simulink model "Mackey-Glass"  (R2020b)
settings: Solver=FixedStepAuto  StartTime=0.0  StopTime=TFinal  FixedStep=0.001  RelTol=1e-3
undefined symbols (not defined in the file or in its folder): coupling, decay_rate, n, nodes
libraries: simulink x1
settings Model: Creator=tian  LastModifiedBy=tian

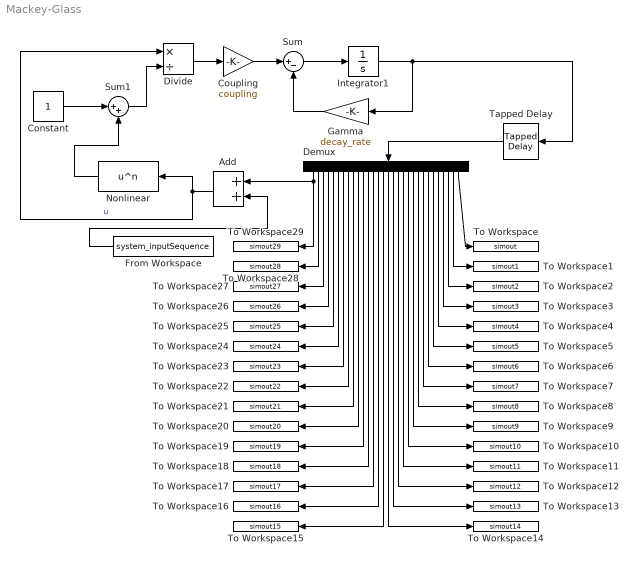
== system Mackey-Glass ==
  Add : Sum
  Constant : Constant
  Coupling : Gain  Gain=coupling
  Demux : Demux  Outputs=30
      settings: DisplayOption=none
  Divide : Product  Inputs=*/
  From Workspace : FromWorkspace  VariableName=system_inputSequence
  Gamma : Gain  Gain=decay_rate
  Integrator1 : Integrator  IgnoreLimit=on
  Nonlinear : Fcn  Expr=u^n
  Sum : Sum  Inputs=|+-
  Sum1 : Sum  Inputs=|++
  Tapped Delay : simulink/Discrete/Tapped Delay  vinit=0.0  samptime=theta  NumDelays=nodes  DelayOrder=Oldest  includeCurrent=off
  To Workspace : ToWorkspace  VariableName=simout  SampleTime=-1
  To Workspace1 : ToWorkspace  VariableName=simout1  SampleTime=-1
  To Workspace10 : ToWorkspace  VariableName=simout10  SampleTime=-1
  To Workspace11 : ToWorkspace  VariableName=simout11  SampleTime=-1
  To Workspace12 : ToWorkspace  VariableName=simout12  SampleTime=-1
  To Workspace13 : ToWorkspace  VariableName=simout13  SampleTime=-1
  To Workspace14 : ToWorkspace  VariableName=simout14  SampleTime=-1
  To Workspace15 : ToWorkspace  VariableName=simout15  SampleTime=-1
  To Workspace16 : ToWorkspace  VariableName=simout16  SampleTime=-1
  To Workspace17 : ToWorkspace  VariableName=simout17  SampleTime=-1
  To Workspace18 : ToWorkspace  VariableName=simout18  SampleTime=-1
  To Workspace19 : ToWorkspace  VariableName=simout19  SampleTime=-1
  To Workspace2 : ToWorkspace  VariableName=simout2  SampleTime=-1
  To Workspace20 : ToWorkspace  VariableName=simout20  SampleTime=-1
  To Workspace21 : ToWorkspace  VariableName=simout21  SampleTime=-1
  To Workspace22 : ToWorkspace  VariableName=simout22  SampleTime=-1
  To Workspace23 : ToWorkspace  VariableName=simout23  SampleTime=-1
  To Workspace24 : ToWorkspace  VariableName=simout24  SampleTime=-1
  To Workspace25 : ToWorkspace  VariableName=simout25  SampleTime=-1
  To Workspace26 : ToWorkspace  VariableName=simout26  SampleTime=-1
  To Workspace27 : ToWorkspace  VariableName=simout27  SampleTime=-1
  To Workspace28 : ToWorkspace  VariableName=simout28  SampleTime=-1
  To Workspace29 : ToWorkspace  VariableName=simout29  SampleTime=-1
  To Workspace3 : ToWorkspace  VariableName=simout3  SampleTime=-1
  To Workspace4 : ToWorkspace  VariableName=simout4  SampleTime=-1
  To Workspace5 : ToWorkspace  VariableName=simout5  SampleTime=-1
  To Workspace6 : ToWorkspace  VariableName=simout6  SampleTime=-1
  To Workspace7 : ToWorkspace  VariableName=simout7  SampleTime=-1
  To Workspace8 : ToWorkspace  VariableName=simout8  SampleTime=-1
  To Workspace9 : ToWorkspace  VariableName=simout9  SampleTime=-1
  wires:
  Demux/5 -> To Workspace25/1
  Demux/21 -> To Workspace9/1
  Demux/25 -> To Workspace5/1
  Demux/29 -> To Workspace1/1
  Demux/10 -> To Workspace20/1
  Demux/20 -> To Workspace10/1
  Demux/23 -> To Workspace7/1
  Demux/7 -> To Workspace23/1
  Demux/22 -> To Workspace8/1
  Demux/19 -> To Workspace11/1
  Demux/17 -> To Workspace13/1
  Demux/18 -> To Workspace12/1
  Demux/15 -> To Workspace15/1
  Demux/14 -> To Workspace16/1
  Demux/16 -> To Workspace14/1
  Nonlinear/1 -> Sum1/2
  Demux/2 -> To Workspace28/1
  Sum1/1 -> Divide/2
  Sum/1 -> Integrator1/1
  Demux/27 -> To Workspace3/1
  Demux/12 -> To Workspace18/1
  Demux/3 -> To Workspace27/1
  Coupling/1 -> Sum/1
  Divide/1 -> Coupling/1
  Constant/1 -> Sum1/1
  Integrator1/1 -> Tapped Delay/1, Gamma/1
  Demux/8 -> To Workspace22/1
  Demux/6 -> To Workspace24/1
  Gamma/1 -> Sum/2
  Demux/24 -> To Workspace6/1
  From Workspace/1 -> Add/2
  Demux/11 -> To Workspace19/1
  Demux/13 -> To Workspace17/1
  Demux/4 -> To Workspace26/1
  Demux/9 -> To Workspace21/1
  Demux/26 -> To Workspace4/1
  Add/1 -> Divide/1, Nonlinear/1  "u"
  Tapped Delay/1 -> Demux/1
  Demux/28 -> To Workspace2/1
  Demux/1 -> Add/1, To Workspace29/1
  Demux/30 -> To Workspace/1
